simulink model "rate_change_filters_txrx_2ch"  (Simulink 8.0)
settings: Solver=VariableStepDiscrete  SolverMode=SingleTasking  StartTime=0.0  StopTime=1e3  RelTol=1e-3
InitFcn:
  | rate_change_filters_init
StartFcn:
  | rate_change_filters_init
values from neighbouring files (symbols this model uses):
  h32_rs = h32    [rate_change_filters_init.m]
  h64_rs = permute(reshape(h64(1:64),4,4,4),[2 1 3])    [rate_change_filters_init.m]
undefined symbols (not defined in the file or in its folder): gcbh, xlBlockLoadCallback, xlGetNormalizedPeriod
libraries: xbsIndex_r4 x519, simulink x4, xbsEDKLib_r4 x1
(part 3 of 4)

== system rate_change_filters_txrx_2ch/Tx Path ==
  2-Ch Interp A : Subsystem
  2-Ch Interp B : Subsystem
  Add : Sum  Inputs=+-
  Add1 : Sum  Inputs=+-
  Chirp : Subsystem
  Chirp1 : Subsystem
  Down Sample{1..4} (4 alike) : xbsIndex_r4/Down Sample  sample_ratio=8  sample_phase="Last Value of Frame  (most efficient)"  en=off  latency=1  dbl_ovrd=off  block_type=dsamp
      settings: xl_area=[8 16 0 0 0 0 0]  block_version=9.1.01
  Integer Delay : Delay  DelayLength=13*2  InputProcessing=Inherited
  Integer Delay1 : Delay  DelayLength=13*2  InputProcessing=Inherited
  Terminator1 : Terminator
  Terminator3 : Terminator
  Tx Scope : Scope  NumInputPorts=8
      settings: TickLabels=on  TimeRange=1000  YMin=-1~-1~-1~-1~-1~-1~-1~-1  YMax=1~1~1~1~1~1~1~1
  TxA_I_10M : xbsIndex_r4/Gateway In  gui_display_data_type=Fixed-point  arith_type="Signed  (2's comp)"  n_bits=16  bin_pt=15  preci_type=Single  exp_width=8  frac_width=24  quantization="Round  (unbiased: +/- Inf)"  overflow=Flag as error  period=1/2  dbl_ovrd=off  timing_constraint=None  locs_specified=off  LOCs={}  UseAsADC=off  ADCChannel='1'  inherit_from_input=off  hdl_port=on  block_type=gatewayin
      settings: infoedit="Gateway in block.  Converts inputs of type Simulink integer, double and fixed point to  Xilinx fixed point type.<P><P>Hardware notes:  In hardware these blocks become top level input ports."  xl_area=[0 0 0 0 16 0 0]  block_version=8.2.01
  TxA_I_40M : xbsIndex_r4/Gateway Out  inherit_from_input=off  hdl_port=on  timing_constraint=None  locs_specified=off  LOCs={}  UseAsDAC=off  DACChannel='1'  block_type=gatewayout
      settings: infoedit="Gateway out block.  Converts Xilinx fixed point inputs into ouputs of type Simulink integer, double, or fixed point.<P><P>Hardware notes:  In hardware these blocks become top level output ports or are discarded, depending on how they are configured."  xl_area=[0 0 0 0 16 0 0]  block_version=8.2.01
  TxA_Q_10M : xbsIndex_r4/Gateway In  gui_display_data_type=Fixed-point  arith_type="Signed  (2's comp)"  n_bits=16  bin_pt=15  preci_type=Single  exp_width=8  frac_width=24  quantization="Round  (unbiased: +/- Inf)"  overflow=Flag as error  period=1/2  dbl_ovrd=off  timing_constraint=None  locs_specified=off  LOCs={}  UseAsADC=off  ADCChannel='1'  inherit_from_input=off  hdl_port=on  block_type=gatewayin
      settings: infoedit="Gateway in block.  Converts inputs of type Simulink integer, double and fixed point to  Xilinx fixed point type.<P><P>Hardware notes:  In hardware these blocks become top level input ports."  xl_area=[0 0 0 0 16 0 0]  block_version=8.2.01
  TxA_Q_40M : xbsIndex_r4/Gateway Out  inherit_from_input=off  hdl_port=on  timing_constraint=None  locs_specified=off  LOCs={}  UseAsDAC=off  DACChannel='1'  block_type=gatewayout
      settings: infoedit="Gateway out block.  Converts Xilinx fixed point inputs into ouputs of type Simulink integer, double, or fixed point.<P><P>Hardware notes:  In hardware these blocks become top level output ports or are discarded, depending on how they are configured."  xl_area=[0 0 0 0 16 0 0]  block_version=8.2.01
  TxB_I_10M : xbsIndex_r4/Gateway In  gui_display_data_type=Fixed-point  arith_type="Signed  (2's comp)"  n_bits=16  bin_pt=15  preci_type=Single  exp_width=8  frac_width=24  quantization="Round  (unbiased: +/- Inf)"  overflow=Flag as error  period=1/2  dbl_ovrd=off  timing_constraint=None  locs_specified=off  LOCs={}  UseAsADC=off  ADCChannel='1'  inherit_from_input=off  hdl_port=on  block_type=gatewayin
      settings: infoedit="Gateway in block.  Converts inputs of type Simulink integer, double and fixed point to  Xilinx fixed point type.<P><P>Hardware notes:  In hardware these blocks become top level input ports."  xl_area=[0 0 0 0 16 0 0]  block_version=8.2.01
  TxB_I_40M : xbsIndex_r4/Gateway Out  inherit_from_input=off  hdl_port=on  timing_constraint=None  locs_specified=off  LOCs={}  UseAsDAC=off  DACChannel='1'  block_type=gatewayout
      settings: infoedit="Gateway out block.  Converts Xilinx fixed point inputs into ouputs of type Simulink integer, double, or fixed point.<P><P>Hardware notes:  In hardware these blocks become top level output ports or are discarded, depending on how they are configured."  xl_area=[0 0 0 0 16 0 0]  block_version=8.2.01
  TxB_Q_10M : xbsIndex_r4/Gateway In  gui_display_data_type=Fixed-point  arith_type="Signed  (2's comp)"  n_bits=16  bin_pt=15  preci_type=Single  exp_width=8  frac_width=24  quantization="Round  (unbiased: +/- Inf)"  overflow=Flag as error  period=1/2  dbl_ovrd=off  timing_constraint=None  locs_specified=off  LOCs={}  UseAsADC=off  ADCChannel='1'  inherit_from_input=off  hdl_port=on  block_type=gatewayin
      settings: infoedit="Gateway in block.  Converts inputs of type Simulink integer, double and fixed point to  Xilinx fixed point type.<P><P>Hardware notes:  In hardware these blocks become top level input ports."  xl_area=[0 0 0 0 16 0 0]  block_version=8.2.01
  TxB_Q_40M : xbsIndex_r4/Gateway Out  inherit_from_input=off  hdl_port=on  timing_constraint=None  locs_specified=off  LOCs={}  UseAsDAC=off  DACChannel='1'  block_type=gatewayout
      settings: infoedit="Gateway out block.  Converts Xilinx fixed point inputs into ouputs of type Simulink integer, double, or fixed point.<P><P>Hardware notes:  In hardware these blocks become top level output ports or are discarded, depending on how they are configured."  xl_area=[0 0 0 0 16 0 0]  block_version=8.2.01
  Up Sample{,1..3} (4 alike) : xbsIndex_r4/Up Sample  sample_ratio=2  copy_samples=on  en=off  latency=0  dbl_ovrd=off  block_type=usamp
      settings: infoedit="Up samples input data.  Inserted values  can be zeros or copies of the most recent input sample.<P><P>Hardware notes: No hardware is needed if inserted values are copies of the input sample; otherwise, a mux and single bit flip-flop are used."  xl_area=[0 0 0 0 0 0 0]  block_version=10.1.3
  wires:
  TxA_I_10M/1 -> Down Sample2/1
  TxA_Q_10M/1 -> Down Sample1/1
  TxB_I_10M/1 -> Down Sample3/1
  TxB_Q_10M/1 -> Down Sample4/1
  Down Sample2/1 -> 2-Ch Interp A/1(XA)
  Chirp/1(Out1) -> TxA_I_10M/1, TxB_I_10M/1, Tx Scope/1
  Integer Delay/1 -> Tx Scope/2, Add/1
  Add/1 -> Tx Scope/4
  Down Sample1/1 -> 2-Ch Interp A/2(XB)
  Chirp1/1(Out1) -> TxA_Q_10M/1, TxB_Q_10M/1, Tx Scope/5
  Add1/1 -> Tx Scope/8
  Down Sample3/1 -> 2-Ch Interp B/1(XA)
  Down Sample4/1 -> 2-Ch Interp B/2(XB)
  2-Ch Interp A/1(YA) -> Up Sample/1
  2-Ch Interp A/2(YB) -> Up Sample1/1
  2-Ch Interp B/1(YA) -> Up Sample2/1
  2-Ch Interp B/2(YB) -> Up Sample3/1
  TxA_I_40M/1 -> Integer Delay/1
  ? -> Tx Scope/3, Add/2
  TxA_Q_40M/1 -> Integer Delay1/1
  Integer Delay1/1 -> Tx Scope/6, Add1/1
  ? -> Tx Scope/7, Add1/2
  TxB_I_40M/1 -> Terminator3/1
  TxB_Q_40M/1 -> Terminator1/1
  Up Sample/1 -> TxA_I_40M/1
  Up Sample1/1 -> TxA_Q_40M/1
  Up Sample2/1 -> TxB_I_40M/1
  Up Sample3/1 -> TxB_Q_40M/1

== system rate_change_filters_txrx_2ch/Control & Coefficients/Rx Coefficients ==
  Addr : Inport
  ROM 0 : xbsIndex_r4/ROM  depth=4  initVector=h64_rs([1:4]+0)  distributed_mem=Distributed memory  rst=off  init_reg=0  en=off  latency=1  gui_display_data_type=Fixed-point  arith_type="Signed  (2's comp)"  n_bits=18  bin_pt=17  preci_type=Single  exp_width=8  frac_width=24  dbl_ovrd=off  optimize=Area  use_rpm=off  block_type=sprom
      settings: xl_area=[9 18 0 18 0 0 0]
  ROM 1 : xbsIndex_r4/ROM  depth=4  initVector=h64_rs([1:4]+4)  distributed_mem=Distributed memory  rst=off  init_reg=0  en=off  latency=1  gui_display_data_type=Fixed-point  arith_type="Signed  (2's comp)"  n_bits=18  bin_pt=17  preci_type=Single  exp_width=8  frac_width=24  dbl_ovrd=off  optimize=Area  use_rpm=off  block_type=sprom
      settings: xl_area=[9 18 0 18 0 0 0]
  ROM 10 : xbsIndex_r4/ROM  depth=4  initVector=h64_rs([1:4]+40)  distributed_mem=Distributed memory  rst=off  init_reg=0  en=off  latency=1  gui_display_data_type=Fixed-point  arith_type="Signed  (2's comp)"  n_bits=18  bin_pt=17  preci_type=Single  exp_width=8  frac_width=24  dbl_ovrd=off  optimize=Area  use_rpm=off  block_type=sprom
      settings: xl_area=[9 18 0 17 0 0 0]
  ROM 11 : xbsIndex_r4/ROM  depth=4  initVector=h64_rs([1:4]+44)  distributed_mem=Distributed memory  rst=off  init_reg=0  en=off  latency=1  gui_display_data_type=Fixed-point  arith_type="Signed  (2's comp)"  n_bits=18  bin_pt=17  preci_type=Single  exp_width=8  frac_width=24  dbl_ovrd=off  optimize=Area  use_rpm=off  block_type=sprom
      settings: xl_area=[9 18 0 17 0 0 0]
  ROM 12 : xbsIndex_r4/ROM  depth=4  initVector=h64_rs([1:4]+48)  distributed_mem=Distributed memory  rst=off  init_reg=0  en=off  latency=1  gui_display_data_type=Fixed-point  arith_type="Signed  (2's comp)"  n_bits=18  bin_pt=17  preci_type=Single  exp_width=8  frac_width=24  dbl_ovrd=off  optimize=Area  use_rpm=off  block_type=sprom
      settings: xl_area=[9 18 0 17 0 0 0]
  ROM 13 : xbsIndex_r4/ROM  depth=4  initVector=h64_rs([1:4]+52)  distributed_mem=Distributed memory  rst=off  init_reg=0  en=off  latency=1  gui_display_data_type=Fixed-point  arith_type="Signed  (2's comp)"  n_bits=18  bin_pt=17  preci_type=Single  exp_width=8  frac_width=24  dbl_ovrd=off  optimize=Area  use_rpm=off  block_type=sprom
      settings: xl_area=[9 18 0 18 0 0 0]
  ROM 14 : xbsIndex_r4/ROM  depth=4  initVector=h64_rs([1:4]+56)  distributed_mem=Distributed memory  rst=off  init_reg=0  en=off  latency=1  gui_display_data_type=Fixed-point  arith_type="Signed  (2's comp)"  n_bits=18  bin_pt=17  preci_type=Single  exp_width=8  frac_width=24  dbl_ovrd=off  optimize=Area  use_rpm=off  block_type=sprom
      settings: xl_area=[9 18 0 18 0 0 0]
  ROM 15 : xbsIndex_r4/ROM  depth=4  initVector=h64_rs([1:4]+60)  distributed_mem=Distributed memory  rst=off  init_reg=0  en=off  latency=1  gui_display_data_type=Fixed-point  arith_type="Signed  (2's comp)"  n_bits=18  bin_pt=17  preci_type=Single  exp_width=8  frac_width=24  dbl_ovrd=off  optimize=Area  use_rpm=off  block_type=sprom
      settings: xl_area=[9 18 0 18 0 0 0]
  ROM 2 : xbsIndex_r4/ROM  depth=4  initVector=h64_rs([1:4]+8)  distributed_mem=Distributed memory  rst=off  init_reg=0  en=off  latency=1  gui_display_data_type=Fixed-point  arith_type="Signed  (2's comp)"  n_bits=18  bin_pt=17  preci_type=Single  exp_width=8  frac_width=24  dbl_ovrd=off  optimize=Area  use_rpm=off  block_type=sprom
      settings: xl_area=[9 18 0 18 0 0 0]
  ROM 3 : xbsIndex_r4/ROM  depth=4  initVector=h64_rs([1:4]+12)  distributed_mem=Distributed memory  rst=off  init_reg=0  en=off  latency=1  gui_display_data_type=Fixed-point  arith_type="Signed  (2's comp)"  n_bits=18  bin_pt=17  preci_type=Single  exp_width=8  frac_width=24  dbl_ovrd=off  optimize=Area  use_rpm=off  block_type=sprom
      settings: xl_area=[9 18 0 17 0 0 0]
  ROM 4 : xbsIndex_r4/ROM  depth=4  initVector=h64_rs([1:4]+16)  distributed_mem=Distributed memory  rst=off  init_reg=0  en=off  latency=1  gui_display_data_type=Fixed-point  arith_type="Signed  (2's comp)"  n_bits=18  bin_pt=17  preci_type=Single  exp_width=8  frac_width=24  dbl_ovrd=off  optimize=Area  use_rpm=off  block_type=sprom
      settings: xl_area=[9 18 0 17 0 0 0]
  ROM 5 : xbsIndex_r4/ROM  depth=4  initVector=h64_rs([1:4]+20)  distributed_mem=Distributed memory  rst=off  init_reg=0  en=off  latency=1  gui_display_data_type=Fixed-point  arith_type="Signed  (2's comp)"  n_bits=18  bin_pt=17  preci_type=Single  exp_width=8  frac_width=24  dbl_ovrd=off  optimize=Area  use_rpm=off  block_type=sprom
      settings: xl_area=[9 18 0 17 0 0 0]
  ROM 6 : xbsIndex_r4/ROM  depth=4  initVector=h64_rs([1:4]+24)  distributed_mem=Distributed memory  rst=off  init_reg=0  en=off  latency=1  gui_display_data_type=Fixed-point  arith_type="Signed  (2's comp)"  n_bits=18  bin_pt=17  preci_type=Single  exp_width=8  frac_width=24  dbl_ovrd=off  optimize=Area  use_rpm=off  block_type=sprom
      settings: xl_area=[9 18 0 18 0 0 0]
  ROM 7 : xbsIndex_r4/ROM  depth=4  initVector=h64_rs([1:4]+28)  distributed_mem=Distributed memory  rst=off  init_reg=0  en=off  latency=1  gui_display_data_type=Fixed-point  arith_type="Signed  (2's comp)"  n_bits=18  bin_pt=17  preci_type=Single  exp_width=8  frac_width=24  dbl_ovrd=off  optimize=Area  use_rpm=off  block_type=sprom
      settings: xl_area=[9 18 0 16 0 0 0]
  ROM 8 : xbsIndex_r4/ROM  depth=4  initVector=h64_rs([1:4]+32)  distributed_mem=Distributed memory  rst=off  init_reg=0  en=off  latency=1  gui_display_data_type=Fixed-point  arith_type="Signed  (2's comp)"  n_bits=18  bin_pt=17  preci_type=Single  exp_width=8  frac_width=24  dbl_ovrd=off  optimize=Area  use_rpm=off  block_type=sprom
      settings: xl_area=[9 18 0 16 0 0 0]
  ROM 9 : xbsIndex_r4/ROM  depth=4  initVector=h64_rs([1:4]+36)  distributed_mem=Distributed memory  rst=off  init_reg=0  en=off  latency=1  gui_display_data_type=Fixed-point  arith_type="Signed  (2's comp)"  n_bits=18  bin_pt=17  preci_type=Single  exp_width=8  frac_width=24  dbl_ovrd=off  optimize=Area  use_rpm=off  block_type=sprom
      settings: xl_area=[9 18 0 18 0 0 0]
  tag scope: ROM_0=global, ROM_10=global, ROM_11=global, ROM_12=global, ROM_13=global, ROM_14=global, ROM_15=global, ROM_1=global, ROM_2=global, ROM_3=global, ROM_4=global, ROM_5=global, ROM_6=global, ROM_7=global, ROM_8=global, ROM_9=global
  wires:
  Addr/1 -> ROM 0/1, ROM 14/1, ROM 15/1, ROM 13/1, ROM 12/1, ROM 11/1, ROM 10/1, ROM 9/1, ROM 8/1, ROM 7/1, ROM 6/1, ROM 5/1, ROM 4/1, ROM 3/1, ROM 2/1, ROM 1/1
  ROM 15/1 -> [ROM_15]
  ROM 14/1 -> [ROM_14]
  ROM 13/1 -> [ROM_13]
  ROM 12/1 -> [ROM_12]
  ROM 11/1 -> [ROM_11]
  ROM 10/1 -> [ROM_10]
  ROM 9/1 -> [ROM_9]
  ROM 8/1 -> [ROM_8]
  ROM 7/1 -> [ROM_7]
  ROM 6/1 -> [ROM_6]
  ROM 5/1 -> [ROM_5]
  ROM 4/1 -> [ROM_4]
  ROM 3/1 -> [ROM_3]
  ROM 2/1 -> [ROM_2]
  ROM 1/1 -> [ROM_1]
  ROM 0/1 -> [ROM_0]

== system rate_change_filters_txrx_2ch/Control & Coefficients/Tx Coefficients ==
  Addr : Inport
  ROM 0 : xbsIndex_r4/ROM  depth=4  initVector=h32_rs([1:4]+0)  distributed_mem=Distributed memory  rst=off  init_reg=0  en=off  latency=1  gui_display_data_type=Fixed-point  arith_type="Signed  (2's comp)"  n_bits=18  bin_pt=17  preci_type=Single  exp_width=8  frac_width=24  dbl_ovrd=off  optimize=Area  use_rpm=off  block_type=sprom
      settings: xl_area=[9 18 0 18 0 0 0]
  ROM 1 : xbsIndex_r4/ROM  depth=4  initVector=h32_rs([1:4]+4)  distributed_mem=Distributed memory  rst=off  init_reg=0  en=off  latency=1  gui_display_data_type=Fixed-point  arith_type="Signed  (2's comp)"  n_bits=18  bin_pt=17  preci_type=Single  exp_width=8  frac_width=24  dbl_ovrd=off  optimize=Area  use_rpm=off  block_type=sprom
      settings: xl_area=[9 18 0 14 0 0 0]
  ROM 2 : xbsIndex_r4/ROM  depth=4  initVector=h32_rs([1:4]+8)  distributed_mem=Distributed memory  rst=off  init_reg=0  en=off  latency=1  gui_display_data_type=Fixed-point  arith_type="Signed  (2's comp)"  n_bits=18  bin_pt=17  preci_type=Single  exp_width=8  frac_width=24  dbl_ovrd=off  optimize=Area  use_rpm=off  block_type=sprom
      settings: xl_area=[9 18 0 17 0 0 0]
  ROM 3 : xbsIndex_r4/ROM  depth=4  initVector=h32_rs([1:4]+12)  distributed_mem=Distributed memory  rst=off  init_reg=0  en=off  latency=1  gui_display_data_type=Fixed-point  arith_type="Signed  (2's comp)"  n_bits=18  bin_pt=17  preci_type=Single  exp_width=8  frac_width=24  dbl_ovrd=off  optimize=Area  use_rpm=off  block_type=sprom
      settings: xl_area=[9 18 0 16 0 0 0]
  ROM 4 : xbsIndex_r4/ROM  depth=4  initVector=h32_rs([1:4]+16)  distributed_mem=Distributed memory  rst=off  init_reg=0  en=off  latency=1  gui_display_data_type=Fixed-point  arith_type="Signed  (2's comp)"  n_bits=18  bin_pt=17  preci_type=Single  exp_width=8  frac_width=24  dbl_ovrd=off  optimize=Area  use_rpm=off  block_type=sprom
      settings: xl_area=[9 18 0 16 0 0 0]
  ROM 5 : xbsIndex_r4/ROM  depth=4  initVector=h32_rs([1:4]+20)  distributed_mem=Distributed memory  rst=off  init_reg=0  en=off  latency=1  gui_display_data_type=Fixed-point  arith_type="Signed  (2's comp)"  n_bits=18  bin_pt=17  preci_type=Single  exp_width=8  frac_width=24  dbl_ovrd=off  optimize=Area  use_rpm=off  block_type=sprom
      settings: xl_area=[9 18 0 17 0 0 0]
  ROM 6 : xbsIndex_r4/ROM  depth=4  initVector=h32_rs([1:4]+24)  distributed_mem=Distributed memory  rst=off  init_reg=0  en=off  latency=1  gui_display_data_type=Fixed-point  arith_type="Signed  (2's comp)"  n_bits=18  bin_pt=17  preci_type=Single  exp_width=8  frac_width=24  dbl_ovrd=off  optimize=Area  use_rpm=off  block_type=sprom
      settings: xl_area=[9 18 0 14 0 0 0]
  ROM 7 : xbsIndex_r4/ROM  depth=4  initVector=h32_rs([1:4]+28)  distributed_mem=Distributed memory  rst=off  init_reg=0  en=off  latency=1  gui_display_data_type=Fixed-point  arith_type="Signed  (2's comp)"  n_bits=18  bin_pt=17  preci_type=Single  exp_width=8  frac_width=24  dbl_ovrd=off  optimize=Area  use_rpm=off  block_type=sprom
      settings: xl_area=[9 18 0 18 0 0 0]
  tag scope: TX_ROM_0=global, TX_ROM_1=global, TX_ROM_2=global, TX_ROM_3=global, TX_ROM_4=global, TX_ROM_5=global, TX_ROM_6=global, TX_ROM_7=global
  wires:
  ROM 0/1 -> [TX_ROM_0]
  ROM 1/1 -> [TX_ROM_1]
  ROM 2/1 -> [TX_ROM_2]
  ROM 3/1 -> [TX_ROM_3]
  ROM 4/1 -> [TX_ROM_4]
  ROM 5/1 -> [TX_ROM_5]
  ROM 6/1 -> [TX_ROM_6]
  ROM 7/1 -> [TX_ROM_7]
  Addr/1 -> ROM 1/1, ROM 2/1, ROM 3/1, ROM 4/1, ROM 5/1, ROM 6/1, ROM 7/1, ROM 0/1

== system rate_change_filters_txrx_2ch/Rx Path/2-Ch Decimation A ==
  note: This convert will overflow, but never for
      | the output samples that are actually
      | captured by the next register.
  note: Need a pipeline stage here to meet 80MHz timing when using non-DSP48 mults in V4.
      | Need double-delays to keep everything lined up
      | when processing two interleaved sample streams.
  XA : Inport
  XB : Inport  Port=2
  Accumulator : xbsIndex_r4/Accumulator  operation=Add  n_bits=32  overflow=Flag as error  scale=1  rst=on  infoeditControl=reset for floating point data type must be asserted for a minimum of 2 cycles  hasbypass=on  en=off  latency=0  dbl_ovrd=off  msb_inp=100  msb=100  lsb=-100  use_behavioral_HDL=on  implementation=Fabric  block_type=accum
      settings: infoedit="Adder or subtractor-based accumulator.   Output type and binary point position match the input.<P><P>Hardware notes: When \"Reinitialize with input 'b' on reset\" is selected, the accumulator is forced to run at the system rate even if the input 'b' is running at a slower rate."  xl_area=[17 33 0 32 0 0 0]  block_version=9.1.01
  Accumulator1 : xbsIndex_r4/Accumulator  operation=Add  n_bits=32  overflow=Flag as error  scale=1  rst=on  infoeditControl=reset for floating point data type must be asserted for a minimum of 2 cycles  hasbypass=on  en=off  latency=0  dbl_ovrd=off  msb_inp=100  msb=100  lsb=-100  use_behavioral_HDL=on  implementation=Fabric  block_type=accum
      settings: infoedit="Adder or subtractor-based accumulator.   Output type and binary point position match the input.<P><P>Hardware notes: When \"Reinitialize with input 'b' on reset\" is selected, the accumulator is forced to run at the system rate even if the input 'b' is running at a slower rate."  xl_area=[17 33 0 32 0 0 0]  block_version=9.1.01
  Adders : Subsystem
  Constant : xbsIndex_r4/Constant  const=3  gui_display_data_type=Fixed-point  arith_type=Unsigned  n_bits=3  bin_pt=0  preci_type=Single  exp_width=8  frac_width=24  explicit_period=off  period=1  equ=P=C  opselect=C  inp2=PCIN>>17  opr=+  inp1=P  carry=CIN  dbl_ovrd=off  block_type=constant
      settings: block_version=9.1.01
  Convert : xbsIndex_r4/Convert  gui_display_data_type=Fixed-point  arith_type="Signed  (2's comp)"  n_bits=14  bin_pt=13  float_type=Single  exp_bits=8  fraction_bits=24  quantization="Round  (unbiased: +/- Inf)"  overflow=Wrap  en=off  latency=0  dbl_ovrd=off  pipeline=off  block_type=convert
      settings: xl_area=[11 0 0 18 0 0 0]  block_version=10.1.3
  Convert1 : xbsIndex_r4/Convert  gui_display_data_type=Fixed-point  arith_type="Signed  (2's comp)"  n_bits=14  bin_pt=13  float_type=Single  exp_bits=8  fraction_bits=24  quantization="Round  (unbiased: +/- Inf)"  overflow=Wrap  en=off  latency=0  dbl_ovrd=off  pipeline=off  block_type=convert
      settings: xl_area=[11 0 0 18 0 0 0]  block_version=10.1.3
  Delay1 : xbsIndex_r4/Delay  rst=off  infoeditControl=Selection of Reset will increase slice count due to use of real FFs and instead of SRLs  en=off  latency=0  dbl_ovrd=off  reg_retiming=off  block_type=delay
      settings: xl_area=[0 0 0 0 0 0 0]  block_version=9.1.01
  Delay16 : xbsIndex_r4/Delay  rst=off  infoeditControl=Selection of Reset will increase slice count due to use of real FFs and instead of SRLs  en=off  latency=0  dbl_ovrd=off  reg_retiming=off  block_type=delay
      settings: xl_area=[0 0 0 0 0 0 0]  block_version=9.1.01
  Delays : Subsystem
  Down Sample : xbsIndex_r4/Down Sample  sample_ratio=4  sample_phase=First Value of Frame  en=off  latency=0  dbl_ovrd=off  block_type=dsamp
      settings: xl_area=[15 15 0 14 0 0 0]  block_version=9.1.01
  Down Sample1 : xbsIndex_r4/Down Sample  sample_ratio=4  sample_phase=First Value of Frame  en=off  latency=0  dbl_ovrd=off  block_type=dsamp
      settings: xl_area=[15 15 0 14 0 0 0]  block_version=9.1.01
  ROMS & Mults : Subsystem
  Register : xbsIndex_r4/Register  init=0  rst=off  en=on  dbl_ovrd=off  block_type=register
      settings: xl_area=[7 14 0 0 0 0 0]  block_version=9.1.01
  Register1 : xbsIndex_r4/Register  init=0  rst=off  en=on  dbl_ovrd=off  block_type=register
      settings: xl_area=[7 14 0 0 0 0 0]  block_version=9.1.01
  Relational : xbsIndex_r4/Relational  mode=a=b  en=off  latency=0  dbl_ovrd=off  block_type=relational
      settings: xl_area=[1 0 0 2 0 0 0]  block_version=9.1.01
  Sample RAMs : Subsystem
  Scale : xbsIndex_r4/Scale  scale_factor=-2  dbl_ovrd=off  block_type=scale
      settings: infoedit=Scales input by a power of two by adjusting the binary point position.<P><P>Hardware notes: In hardware this block costs nothing.  block_version=10.1.3
  Scale1 : xbsIndex_r4/Scale  scale_factor=-2  dbl_ovrd=off  block_type=scale
      settings: infoedit=Scales input by a power of two by adjusting the binary point position.<P><P>Hardware notes: In hardware this block costs nothing.  block_version=10.1.3
  TDD : xbsIndex_r4/Time Division Demultiplexer  frame_pattern=ones(1,2)  impl_style=Multiple Channel  vin=off  dbl_ovrd=off  explicit_period=off  period=1  block_type=tdd
      settings: infoedit=Samples presented at the input are selected and down-sampled according to the frame sampling pattern specified. The sampled input is presented either as a single or multiple channel at the output.  xl_area=[42 84 0 0 0 0 0]  block_version=9.1.01
  YA : Outport
  YB : Outport  Port=2
  wires:
  ROMS & Mults/8(Out8) -> Adders/8(In8)
  ROMS & Mults/7(Out7) -> Adders/7(In7)
  ROMS & Mults/6(Out6) -> Adders/6(In6)
  ROMS & Mults/5(Out5) -> Adders/5(In5)
  ROMS & Mults/4(Out4) -> Adders/4(In4)
  ROMS & Mults/3(Out3) -> Adders/3(In3)
  ROMS & Mults/2(Out2) -> Adders/2(In2)
  ROMS & Mults/1(Out1) -> Adders/1(In1)
  ROMS & Mults/16(Out16) -> Adders/16(In16)
  ROMS & Mults/15(Out15) -> Adders/15(In15)
  ROMS & Mults/14(Out14) -> Adders/14(In14)
  ROMS & Mults/13(Out13) -> Adders/13(In13)
  ROMS & Mults/12(Out12) -> Adders/12(In12)
  ROMS & Mults/11(Out11) -> Adders/11(In11)
  ROMS & Mults/10(Out10) -> Adders/10(In10)
  ROMS & Mults/9(Out9) -> Adders/9(In9)
  Register/1 -> Down Sample/1
  Down Sample/1 -> YB/1
  Constant/1 -> Relational/1
  Accumulator/1 -> Scale/1
  [CoefAddr] -> Delay16/1, Delay1/1
  Scale/1 -> Convert/1
  Convert/1 -> Register/1
  XA/1 -> Sample RAMs/1(XA)
  XB/1 -> Sample RAMs/2(XB)
  Accumulator1/1 -> Scale1/1
  Scale1/1 -> Convert1/1
  Convert1/1 -> Register1/1
  Register1/1 -> Down Sample1/1
  Down Sample1/1 -> YA/1
  Adders/1(Out1) -> TDD/1
  TDD/1 -> Accumulator1/1
  TDD/2 -> Accumulator/1
  Relational/1 -> Accumulator1/2, Accumulator/2, Register1/2, Register/2
  Sample RAMs/1(Out1) -> Delays/1(In1)
  Sample RAMs/2(Out2) -> Delays/2(In2)
  Sample RAMs/3(Out3) -> Delays/3(In3)
  Sample RAMs/4(Out4) -> Delays/4(In4)
  Sample RAMs/5(Out5) -> Delays/5(In5)
  Sample RAMs/6(Out6) -> Delays/6(In6)
  Sample RAMs/7(Out7) -> Delays/7(In7)
  Sample RAMs/8(Out8) -> Delays/8(In8)
  Sample RAMs/9(Out9) -> Delays/9(In9)
  Sample RAMs/10(Out10) -> Delays/10(In10)
  Sample RAMs/11(Out11) -> Delays/11(In11)
  Sample RAMs/12(Out12) -> Delays/12(In12)
  Sample RAMs/13(Out13) -> Delays/13(In13)
  Sample RAMs/14(Out14) -> Delays/14(In14)
  Sample RAMs/15(Out15) -> Delays/15(In15)
  Sample RAMs/16(Out16) -> Delays/16(In16)
  Delay16/1 -> Sample RAMs/3(Addr)
  Delay1/1 -> Relational/2
  Delays/1(Out1) -> ROMS & Mults/1(In1)
  Delays/2(Out2) -> ROMS & Mults/2(In2)
  Delays/3(Out3) -> ROMS & Mults/3(In3)
  Delays/4(Out4) -> ROMS & Mults/4(In4)
  Delays/5(Out5) -> ROMS & Mults/5(In5)
  Delays/6(Out6) -> ROMS & Mults/6(In6)
  Delays/7(Out7) -> ROMS & Mults/7(In7)
  Delays/8(Out8) -> ROMS & Mults/8(In8)
  Delays/9(Out9) -> ROMS & Mults/9(In9)
  Delays/10(Out10) -> ROMS & Mults/10(In10)
  Delays/11(Out11) -> ROMS & Mults/11(In11)
  Delays/12(Out12) -> ROMS & Mults/12(In12)
  Delays/13(Out13) -> ROMS & Mults/13(In13)
  Delays/14(Out14) -> ROMS & Mults/14(In14)
  Delays/15(Out15) -> ROMS & Mults/15(In15)
  Delays/16(Out16) -> ROMS & Mults/16(In16)

== system rate_change_filters_txrx_2ch/Rx Path/2-Ch Decimation B ==
  note: Need a pipeline stage here to meet 80MHz timing when using non-DSP48 mults in V4.
      | Need double-delays to keep everything lined up
      | when processing two interleaved sample streams.
  note: This convert will overflow, but never for
      | the output samples that are actually
      | captured by the next register.
  XA : Inport
  XB : Inport  Port=2
  Accumulator : xbsIndex_r4/Accumulator  operation=Add  n_bits=32  overflow=Flag as error  scale=1  rst=on  infoeditControl=reset for floating point data type must be asserted for a minimum of 2 cycles  hasbypass=on  en=off  latency=0  dbl_ovrd=off  msb_inp=100  msb=100  lsb=-100  use_behavioral_HDL=on  implementation=Fabric  block_type=accum
      settings: infoedit="Adder or subtractor-based accumulator.   Output type and binary point position match the input.<P><P>Hardware notes: When \"Reinitialize with input 'b' on reset\" is selected, the accumulator is forced to run at the system rate even if the input 'b' is running at a slower rate."  xl_area=[17 33 0 32 0 0 0]  block_version=9.1.01
  Accumulator1 : xbsIndex_r4/Accumulator  operation=Add  n_bits=32  overflow=Flag as error  scale=1  rst=on  infoeditControl=reset for floating point data type must be asserted for a minimum of 2 cycles  hasbypass=on  en=off  latency=0  dbl_ovrd=off  msb_inp=100  msb=100  lsb=-100  use_behavioral_HDL=on  implementation=Fabric  block_type=accum
      settings: infoedit="Adder or subtractor-based accumulator.   Output type and binary point position match the input.<P><P>Hardware notes: When \"Reinitialize with input 'b' on reset\" is selected, the accumulator is forced to run at the system rate even if the input 'b' is running at a slower rate."  xl_area=[17 33 0 32 0 0 0]  block_version=9.1.01
  Adders : Subsystem
  Constant : xbsIndex_r4/Constant  const=3  gui_display_data_type=Fixed-point  arith_type=Unsigned  n_bits=3  bin_pt=0  preci_type=Single  exp_width=8  frac_width=24  explicit_period=off  period=1  equ=P=C  opselect=C  inp2=PCIN>>17  opr=+  inp1=P  carry=CIN  dbl_ovrd=off  block_type=constant
      settings: block_version=9.1.01
  Convert : xbsIndex_r4/Convert  gui_display_data_type=Fixed-point  arith_type="Signed  (2's comp)"  n_bits=14  bin_pt=13  float_type=Single  exp_bits=8  fraction_bits=24  quantization="Round  (unbiased: +/- Inf)"  overflow=Wrap  en=off  latency=0  dbl_ovrd=off  pipeline=off  block_type=convert
      settings: xl_area=[11 0 0 18 0 0 0]  block_version=10.1.3
  Convert1 : xbsIndex_r4/Convert  gui_display_data_type=Fixed-point  arith_type="Signed  (2's comp)"  n_bits=14  bin_pt=13  float_type=Single  exp_bits=8  fraction_bits=24  quantization="Round  (unbiased: +/- Inf)"  overflow=Wrap  en=off  latency=0  dbl_ovrd=off  pipeline=off  block_type=convert
      settings: xl_area=[11 0 0 18 0 0 0]  block_version=10.1.3
  Delay1 : xbsIndex_r4/Delay  rst=off  infoeditControl=Selection of Reset will increase slice count due to use of real FFs and instead of SRLs  en=off  latency=0  dbl_ovrd=off  reg_retiming=off  block_type=delay
      settings: xl_area=[0 0 0 0 0 0 0]  block_version=9.1.01
  Delay16 : xbsIndex_r4/Delay  rst=off  infoeditControl=Selection of Reset will increase slice count due to use of real FFs and instead of SRLs  en=off  latency=0  dbl_ovrd=off  reg_retiming=off  block_type=delay
      settings: xl_area=[0 0 0 0 0 0 0]  block_version=9.1.01
  Delays : Subsystem
  Down Sample : xbsIndex_r4/Down Sample  sample_ratio=4  sample_phase=First Value of Frame  en=off  latency=0  dbl_ovrd=off  block_type=dsamp
      settings: xl_area=[15 15 0 14 0 0 0]  block_version=9.1.01
  Down Sample1 : xbsIndex_r4/Down Sample  sample_ratio=4  sample_phase=First Value of Frame  en=off  latency=0  dbl_ovrd=off  block_type=dsamp
      settings: xl_area=[15 15 0 14 0 0 0]  block_version=9.1.01
  ROMS & Mults : Subsystem
  Register : xbsIndex_r4/Register  init=0  rst=off  en=on  dbl_ovrd=off  block_type=register
      settings: xl_area=[7 14 0 0 0 0 0]  block_version=9.1.01
  Register1 : xbsIndex_r4/Register  init=0  rst=off  en=on  dbl_ovrd=off  block_type=register
      settings: xl_area=[7 14 0 0 0 0 0]  block_version=9.1.01
  Relational : xbsIndex_r4/Relational  mode=a=b  en=off  latency=0  dbl_ovrd=off  block_type=relational
      settings: xl_area=[1 0 0 2 0 0 0]  block_version=9.1.01
  Sample RAMs : Subsystem
  Scale : xbsIndex_r4/Scale  scale_factor=-2  dbl_ovrd=off  block_type=scale
      settings: infoedit=Scales input by a power of two by adjusting the binary point position.<P><P>Hardware notes: In hardware this block costs nothing.  block_version=10.1.3
  Scale1 : xbsIndex_r4/Scale  scale_factor=-2  dbl_ovrd=off  block_type=scale
      settings: infoedit=Scales input by a power of two by adjusting the binary point position.<P><P>Hardware notes: In hardware this block costs nothing.  block_version=10.1.3
  TDD : xbsIndex_r4/Time Division Demultiplexer  frame_pattern=ones(1,2)  impl_style=Multiple Channel  vin=off  dbl_ovrd=off  explicit_period=off  period=1  block_type=tdd
      settings: infoedit=Samples presented at the input are selected and down-sampled according to the frame sampling pattern specified. The sampled input is presented either as a single or multiple channel at the output.  xl_area=[42 84 0 0 0 0 0]  block_version=9.1.01
  YA : Outport
  YB : Outport  Port=2
  wires:
  Delays/16(Out16) -> ROMS & Mults/16(In16)
  Delays/15(Out15) -> ROMS & Mults/15(In15)
  Delays/14(Out14) -> ROMS & Mults/14(In14)
  Delays/13(Out13) -> ROMS & Mults/13(In13)
  Delays/12(Out12) -> ROMS & Mults/12(In12)
  Delays/11(Out11) -> ROMS & Mults/11(In11)
  Delays/10(Out10) -> ROMS & Mults/10(In10)
  Delays/9(Out9) -> ROMS & Mults/9(In9)
  Delays/8(Out8) -> ROMS & Mults/8(In8)
  Delays/7(Out7) -> ROMS & Mults/7(In7)
  Delays/6(Out6) -> ROMS & Mults/6(In6)
  Delays/5(Out5) -> ROMS & Mults/5(In5)
  Delays/4(Out4) -> ROMS & Mults/4(In4)
  Delays/3(Out3) -> ROMS & Mults/3(In3)
  Delays/2(Out2) -> ROMS & Mults/2(In2)
  Delays/1(Out1) -> ROMS & Mults/1(In1)
  Delay1/1 -> Relational/2
  Delay16/1 -> Sample RAMs/3(Addr)
  Sample RAMs/16(Out16) -> Delays/16(In16)
  Sample RAMs/15(Out15) -> Delays/15(In15)
  Sample RAMs/14(Out14) -> Delays/14(In14)
  Sample RAMs/13(Out13) -> Delays/13(In13)
  Sample RAMs/12(Out12) -> Delays/12(In12)
  Sample RAMs/11(Out11) -> Delays/11(In11)
  Sample RAMs/10(Out10) -> Delays/10(In10)
  Sample RAMs/9(Out9) -> Delays/9(In9)
  Sample RAMs/8(Out8) -> Delays/8(In8)
  Sample RAMs/7(Out7) -> Delays/7(In7)
  Sample RAMs/6(Out6) -> Delays/6(In6)
  Sample RAMs/5(Out5) -> Delays/5(In5)
  Sample RAMs/4(Out4) -> Delays/4(In4)
  Sample RAMs/3(Out3) -> Delays/3(In3)
  Sample RAMs/2(Out2) -> Delays/2(In2)
  Sample RAMs/1(Out1) -> Delays/1(In1)
  Relational/1 -> Register/2, Register1/2, Accumulator/2, Accumulator1/2
  TDD/2 -> Accumulator/1
  TDD/1 -> Accumulator1/1
  Adders/1(Out1) -> TDD/1
  Down Sample1/1 -> YA/1
  Register1/1 -> Down Sample1/1
  Convert1/1 -> Register1/1
  Scale1/1 -> Convert1/1
  Accumulator1/1 -> Scale1/1
  XB/1 -> Sample RAMs/2(XB)
  XA/1 -> Sample RAMs/1(XA)
  Convert/1 -> Register/1
  Scale/1 -> Convert/1
  [CoefAddr] -> Delay1/1, Delay16/1
  Accumulator/1 -> Scale/1
  Constant/1 -> Relational/1
  Down Sample/1 -> YB/1
  Register/1 -> Down Sample/1
  ROMS & Mults/9(Out9) -> Adders/9(In9)
  ROMS & Mults/10(Out10) -> Adders/10(In10)
  ROMS & Mults/11(Out11) -> Adders/11(In11)
  ROMS & Mults/12(Out12) -> Adders/12(In12)
  ROMS & Mults/13(Out13) -> Adders/13(In13)
  ROMS & Mults/14(Out14) -> Adders/14(In14)
  ROMS & Mults/15(Out15) -> Adders/15(In15)
  ROMS & Mults/16(Out16) -> Adders/16(In16)
  ROMS & Mults/1(Out1) -> Adders/1(In1)
  ROMS & Mults/2(Out2) -> Adders/2(In2)
  ROMS & Mults/3(Out3) -> Adders/3(In3)
  ROMS & Mults/4(Out4) -> Adders/4(In4)
  ROMS & Mults/5(Out5) -> Adders/5(In5)
  ROMS & Mults/6(Out6) -> Adders/6(In6)
  ROMS & Mults/7(Out7) -> Adders/7(In7)
  ROMS & Mults/8(Out8) -> Adders/8(In8)

== system rate_change_filters_txrx_2ch/Rx Path/Chirp ==
  Chirp Signal : simulink/Sources/Chirp Signal  f1=0  T=512  f2=0.5
  Gain : Gain  Gain=0.99
  Out1 : Outport
  wires:
  Chirp Signal/1 -> Gain/1
  Gain/1 -> Out1/1

== system rate_change_filters_txrx_2ch/Rx Path/Chirp1 ==
  Chirp Signal : simulink/Sources/Chirp Signal  f1=0  T=512  f2=0.5
  Gain : Gain  Gain=-0.99
  Out1 : Outport
  wires:
  Gain/1 -> Out1/1
  Chirp Signal/1 -> Gain/1

== system rate_change_filters_txrx_2ch/Tx Path/2-Ch Interp A ==
  XA : Inport
  XB : Inport  Port=2
  Adders : Subsystem
  Mults & ROMs : Subsystem
  Sample RAMs : Subsystem
  TDD : xbsIndex_r4/Time Division Demultiplexer  frame_pattern=ones(1,2)  impl_style=Multiple Channel  vin=off  dbl_ovrd=off  explicit_period=off  period=1  block_type=tdd
      settings: infoedit=Samples presented at the input are selected and down-sampled according to the frame sampling pattern specified. The sampled input is presented either as a single or multiple channel at the output.  xl_area=[24 48 0 0 0 0 0]  block_version=9.1.01
  YA : Outport
  YB : Outport  Port=2
  wires:
  Mults & ROMs/8(Out8) -> Adders/8(In8)
  Mults & ROMs/7(Out7) -> Adders/7(In7)
  Mults & ROMs/6(Out6) -> Adders/6(In6)
  Mults & ROMs/5(Out5) -> Adders/5(In5)
  Mults & ROMs/4(Out4) -> Adders/4(In4)
  Mults & ROMs/3(Out3) -> Adders/3(In3)
  Mults & ROMs/2(Out2) -> Adders/2(In2)
  Mults & ROMs/1(Out1) -> Adders/1(In1)
  XA/1 -> Sample RAMs/1(A)
  XB/1 -> Sample RAMs/2(B)
  Sample RAMs/1(Out1) -> Mults & ROMs/1(In1)
  Sample RAMs/2(Out2) -> Mults & ROMs/2(In2)
  Sample RAMs/3(Out3) -> Mults & ROMs/3(In3)
  Sample RAMs/4(Out4) -> Mults & ROMs/4(In4)
  Sample RAMs/5(Out5) -> Mults & ROMs/5(In5)
  Sample RAMs/6(Out6) -> Mults & ROMs/6(In6)
  Sample RAMs/7(Out7) -> Mults & ROMs/7(In7)
  Sample RAMs/8(Out8) -> Mults & ROMs/8(In8)
  Adders/1(Out1) -> TDD/1
  TDD/1 -> YA/1
  TDD/2 -> YB/1

== system rate_change_filters_txrx_2ch/Tx Path/2-Ch Interp B ==
  XA : Inport
  XB : Inport  Port=2
  Adders : Subsystem
  Mults & ROMs : Subsystem
  Sample RAMs : Subsystem
  TDD : xbsIndex_r4/Time Division Demultiplexer  frame_pattern=ones(1,2)  impl_style=Multiple Channel  vin=off  dbl_ovrd=off  explicit_period=off  period=1  block_type=tdd
      settings: infoedit=Samples presented at the input are selected and down-sampled according to the frame sampling pattern specified. The sampled input is presented either as a single or multiple channel at the output.  xl_area=[24 48 0 0 0 0 0]  block_version=9.1.01
  YA : Outport
  YB : Outport  Port=2
  wires:
  TDD/2 -> YB/1
  TDD/1 -> YA/1
  Adders/1(Out1) -> TDD/1
  Sample RAMs/8(Out8) -> Mults & ROMs/8(In8)
  Sample RAMs/7(Out7) -> Mults & ROMs/7(In7)
  Sample RAMs/6(Out6) -> Mults & ROMs/6(In6)
  Sample RAMs/5(Out5) -> Mults & ROMs/5(In5)
  Sample RAMs/4(Out4) -> Mults & ROMs/4(In4)
  Sample RAMs/3(Out3) -> Mults & ROMs/3(In3)
  Sample RAMs/2(Out2) -> Mults & ROMs/2(In2)
  Sample RAMs/1(Out1) -> Mults & ROMs/1(In1)
  XB/1 -> Sample RAMs/2(B)
  XA/1 -> Sample RAMs/1(A)
  Mults & ROMs/1(Out1) -> Adders/1(In1)
  Mults & ROMs/2(Out2) -> Adders/2(In2)
  Mults & ROMs/3(Out3) -> Adders/3(In3)
  Mults & ROMs/4(Out4) -> Adders/4(In4)
  Mults & ROMs/5(Out5) -> Adders/5(In5)
  Mults & ROMs/6(Out6) -> Adders/6(In6)
  Mults & ROMs/7(Out7) -> Adders/7(In7)
  Mults & ROMs/8(Out8) -> Adders/8(In8)

== system rate_change_filters_txrx_2ch/Tx Path/Chirp ==
  Chirp Signal : simulink/Sources/Chirp Signal  f1=0  T=512  f2=0.5
  Gain : Gain  Gain=0.95
  Out1 : Outport
  wires:
  Chirp Signal/1 -> Gain/1
  Gain/1 -> Out1/1

== system rate_change_filters_txrx_2ch/Tx Path/Chirp1 ==
  Chirp Signal : simulink/Sources/Chirp Signal  f1=0  T=512  f2=0.5
  Gain : Gain  Gain=-0.95
  Out1 : Outport
  wires:
  Gain/1 -> Out1/1
  Chirp Signal/1 -> Gain/1

== system rate_change_filters_txrx_2ch/Rx Path/2-Ch Decimation A/Adders ==
  In1 : Inport
  In2 : Inport  Port=2
  In3 : Inport  Port=3
  In4 : Inport  Port=4
  In5 : Inport  Port=5
  In6 : Inport  Port=6
  In7 : Inport  Port=7
  In8 : Inport  Port=8
  In9 : Inport  Port=9
  In10 : Inport  Port=10
  In11 : Inport  Port=11
  In12 : Inport  Port=12
  In13 : Inport  Port=13
  In14 : Inport  Port=14
  In15 : Inport  Port=15
  In16 : Inport  Port=16
  AddSub6 : xbsIndex_r4/AddSub  mode=Addition  use_carryin=off  use_carryout=off  en=off  latency=0  precision=Full  arith_type="Signed  (2's comp)"  n_bits=1  bin_pt=0  quantization=Truncate  overflow=Flag as error  dbl_ovrd=off  use_behavioral_HDL=on  hw_selection=Fabric  pipelined=off  use_rpm=on  block_type=addsub
      settings: xl_area=[15 0 0 28 0 0 0]  block_version=9.1.01
  Adder Tree : Subsystem
  Adder Tree1 : Subsystem
  Out1 : Outport
  wires:
  Adder Tree/1(Out1) -> AddSub6/2
  Adder Tree1/1(Out1) -> AddSub6/1
  In1/1 -> Adder Tree1/1(In1)
  In2/1 -> Adder Tree1/2(In2)
  In3/1 -> Adder Tree1/3(In3)
  In4/1 -> Adder Tree1/4(In4)
  In5/1 -> Adder Tree1/5(In5)
  In6/1 -> Adder Tree1/6(In6)
  In7/1 -> Adder Tree1/7(In7)
  In8/1 -> Adder Tree1/8(In8)
  In9/1 -> Adder Tree/1(In1)
  In10/1 -> Adder Tree/2(In2)
  In11/1 -> Adder Tree/3(In3)
  In12/1 -> Adder Tree/4(In4)
  AddSub6/1 -> Out1/1
  In13/1 -> Adder Tree/5(In5)
  In14/1 -> Adder Tree/6(In6)
  In15/1 -> Adder Tree/7(In7)
  In16/1 -> Adder Tree/8(In8)

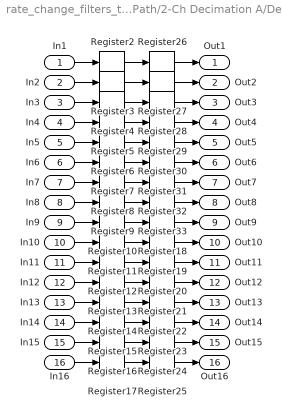
== system rate_change_filters_txrx_2ch/Rx Path/2-Ch Decimation A/Delays ==
  In1 : Inport
  In2 : Inport  Port=2
  In3 : Inport  Port=3
  In4 : Inport  Port=4
  In5 : Inport  Port=5
  In6 : Inport  Port=6
  In7 : Inport  Port=7
  In8 : Inport  Port=8
  In9 : Inport  Port=9
  In10 : Inport  Port=10
  In11 : Inport  Port=11
  In12 : Inport  Port=12
  In13 : Inport  Port=13
  In14 : Inport  Port=14
  In15 : Inport  Port=15
  In16 : Inport  Port=16
  Register{2..33} (32 alike) : xbsIndex_r4/Register  init=0  rst=off  en=off  dbl_ovrd=off  block_type=register
      settings: xl_area=[7 14 0 0 0 0 0]
  Out1 : Outport
  Out2 : Outport  Port=2
  Out3 : Outport  Port=3
  Out4 : Outport  Port=4
  Out5 : Outport  Port=5
  Out6 : Outport  Port=6
  Out7 : Outport  Port=7
  Out8 : Outport  Port=8
  Out9 : Outport  Port=9
  Out10 : Outport  Port=10
  Out11 : Outport  Port=11
  Out12 : Outport  Port=12
  Out13 : Outport  Port=13
  Out14 : Outport  Port=14
  Out15 : Outport  Port=15
  Out16 : Outport  Port=16
  wires:
  Register2/1 -> Register26/1
  Register3/1 -> Register27/1
  Register4/1 -> Register28/1
  Register5/1 -> Register29/1
  Register6/1 -> Register30/1
  Register7/1 -> Register31/1
  Register8/1 -> Register32/1
  Register9/1 -> Register33/1
  Register10/1 -> Register18/1
  Register11/1 -> Register19/1
  Register12/1 -> Register20/1
  Register13/1 -> Register21/1
  Register14/1 -> Register22/1
  Register15/1 -> Register23/1
  Register16/1 -> Register24/1
  Register17/1 -> Register25/1
  In1/1 -> Register2/1
  Register26/1 -> Out1/1
  Register27/1 -> Out2/1
  In2/1 -> Register3/1
  Register28/1 -> Out3/1
  In3/1 -> Register4/1
  Register29/1 -> Out4/1
  In4/1 -> Register5/1
  Register30/1 -> Out5/1
  In5/1 -> Register6/1
  Register31/1 -> Out6/1
  In6/1 -> Register7/1
  Register32/1 -> Out7/1
  In7/1 -> Register8/1
  Register33/1 -> Out8/1
  In8/1 -> Register9/1
  In9/1 -> Register10/1
  Register18/1 -> Out9/1
  In10/1 -> Register11/1
  Register19/1 -> Out10/1
  In11/1 -> Register12/1
  Register20/1 -> Out11/1
  In12/1 -> Register13/1
  Register21/1 -> Out12/1
  In13/1 -> Register14/1
  Register22/1 -> Out13/1
  In14/1 -> Register15/1
  Register23/1 -> Out14/1
  In15/1 -> Register16/1
  Register24/1 -> Out15/1
  In16/1 -> Register17/1
  Register25/1 -> Out16/1

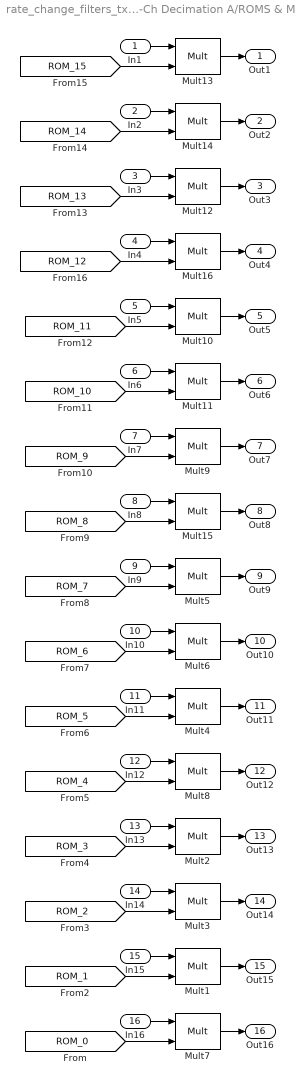
== system rate_change_filters_txrx_2ch/Rx Path/2-Ch Decimation A/ROMS & Mults ==
  In1 : Inport
  In2 : Inport  Port=2
  In3 : Inport  Port=3
  In4 : Inport  Port=4
  In5 : Inport  Port=5
  In6 : Inport  Port=6
  In7 : Inport  Port=7
  In8 : Inport  Port=8
  In9 : Inport  Port=9
  In10 : Inport  Port=10
  In11 : Inport  Port=11
  In12 : Inport  Port=12
  In13 : Inport  Port=13
  In14 : Inport  Port=14
  In15 : Inport  Port=15
  In16 : Inport  Port=16
  Mult{1..16} (16 alike) : xbsIndex_r4/Mult  precision=User Defined  arith_type="Signed  (2's comp)"  n_bits=24  bin_pt=22  quantization=Truncate  overflow=Flag as error  en=off  latency=1  dbl_ovrd=off  use_behavioral_HDL=off  opt=Speed  use_embedded=on  optimum_pipeline=off  pipeline=off  use_rpm=on  placement_style=Rectangular shape  block_type=mult
      settings: infoedit=Hardware notes: To use the internal pipeline stage of the dedicated multiplier you must select 'Pipeline for maximum performance'.  xl_area=[16 32 0 32 0 1 0]  block_version=9.1.01
  Out1 : Outport
  Out2 : Outport  Port=2
  Out3 : Outport  Port=3
  Out4 : Outport  Port=4
  Out5 : Outport  Port=5
  Out6 : Outport  Port=6
  Out7 : Outport  Port=7
  Out8 : Outport  Port=8
  Out9 : Outport  Port=9
  Out10 : Outport  Port=10
  Out11 : Outport  Port=11
  Out12 : Outport  Port=12
  Out13 : Outport  Port=13
  Out14 : Outport  Port=14
  Out15 : Outport  Port=15
  Out16 : Outport  Port=16
  wires:
  [ROM_15] -> Mult13/2
  [ROM_14] -> Mult14/2
  [ROM_13] -> Mult12/2
  [ROM_12] -> Mult16/2
  [ROM_11] -> Mult10/2
  [ROM_10] -> Mult11/2
  [ROM_9] -> Mult9/2
  [ROM_8] -> Mult15/2
  [ROM_7] -> Mult5/2
  [ROM_6] -> Mult6/2
  [ROM_5] -> Mult4/2
  [ROM_4] -> Mult8/2
  [ROM_3] -> Mult2/2
  [ROM_2] -> Mult3/2
  [ROM_1] -> Mult1/2
  [ROM_0] -> Mult7/2
  In1/1 -> Mult13/1
  Mult13/1 -> Out1/1
  In2/1 -> Mult14/1
  Mult14/1 -> Out2/1
  In3/1 -> Mult12/1
  Mult12/1 -> Out3/1
  In4/1 -> Mult16/1
  Mult16/1 -> Out4/1
  In5/1 -> Mult10/1
  Mult10/1 -> Out5/1
  In6/1 -> Mult11/1
  Mult11/1 -> Out6/1
  In7/1 -> Mult9/1
  Mult9/1 -> Out7/1
  In8/1 -> Mult15/1
  Mult15/1 -> Out8/1
  In9/1 -> Mult5/1
  Mult5/1 -> Out9/1
  In10/1 -> Mult6/1
  Mult6/1 -> Out10/1
  In11/1 -> Mult4/1
  Mult4/1 -> Out11/1
  In12/1 -> Mult8/1
  Mult8/1 -> Out12/1
  In13/1 -> Mult2/1
  Mult2/1 -> Out13/1
  In14/1 -> Mult3/1
  Mult3/1 -> Out14/1
  In15/1 -> Mult1/1
  Mult1/1 -> Out15/1
  In16/1 -> Mult7/1
  Mult7/1 -> Out16/1

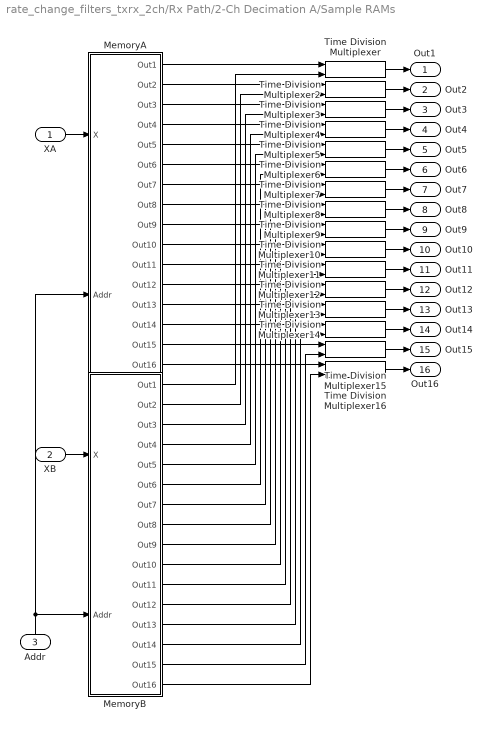
== system rate_change_filters_txrx_2ch/Rx Path/2-Ch Decimation A/Sample RAMs ==
  XA : Inport
  XB : Inport  Port=2
  Addr : Inport  Port=3
  MemoryA : Subsystem
  MemoryB : Subsystem
  Time Division Multiplexer{,2..16} (16 alike) : xbsIndex_r4/Time Division Multiplexer  inputs=2  vin=off  dbl_ovrd=off  explicit_period=off  period=1  block_type=tdm
      settings: infoedit="Multiple inputs are sampled and  presented serially at the output."  xl_area=[3 2 0 31 0 0 0]  block_version=10.1.3
  Out1 : Outport
  Out2 : Outport  Port=2
  Out3 : Outport  Port=3
  Out4 : Outport  Port=4
  Out5 : Outport  Port=5
  Out6 : Outport  Port=6
  Out7 : Outport  Port=7
  Out8 : Outport  Port=8
  Out9 : Outport  Port=9
  Out10 : Outport  Port=10
  Out11 : Outport  Port=11
  Out12 : Outport  Port=12
  Out13 : Outport  Port=13
  Out14 : Outport  Port=14
  Out15 : Outport  Port=15
  Out16 : Outport  Port=16
  wires:
  Addr/1 -> MemoryA/2(Addr), MemoryB/2(Addr)
  MemoryA/1(Out1) -> Time Division Multiplexer/1
  MemoryA/2(Out2) -> Time Division Multiplexer2/1
  MemoryA/3(Out3) -> Time Division Multiplexer3/1
  MemoryA/4(Out4) -> Time Division Multiplexer4/1
  MemoryA/5(Out5) -> Time Division Multiplexer5/1
  MemoryA/6(Out6) -> Time Division Multiplexer6/1
  MemoryA/7(Out7) -> Time Division Multiplexer7/1
  MemoryA/8(Out8) -> Time Division Multiplexer8/1
  MemoryA/9(Out9) -> Time Division Multiplexer9/1
  MemoryA/10(Out10) -> Time Division Multiplexer10/1
  MemoryA/11(Out11) -> Time Division Multiplexer11/1
  MemoryA/12(Out12) -> Time Division Multiplexer12/1
  MemoryA/13(Out13) -> Time Division Multiplexer13/1
  MemoryA/14(Out14) -> Time Division Multiplexer14/1
  MemoryA/15(Out15) -> Time Division Multiplexer15/1
  MemoryA/16(Out16) -> Time Division Multiplexer16/1
  MemoryB/1(Out1) -> Time Division Multiplexer/2
  MemoryB/2(Out2) -> Time Division Multiplexer2/2
  MemoryB/3(Out3) -> Time Division Multiplexer3/2
  MemoryB/4(Out4) -> Time Division Multiplexer4/2
  MemoryB/5(Out5) -> Time Division Multiplexer5/2
  MemoryB/6(Out6) -> Time Division Multiplexer6/2
  MemoryB/7(Out7) -> Time Division Multiplexer7/2
  MemoryB/8(Out8) -> Time Division Multiplexer8/2
  MemoryB/9(Out9) -> Time Division Multiplexer9/2
  MemoryB/10(Out10) -> Time Division Multiplexer10/2
  MemoryB/11(Out11) -> Time Division Multiplexer11/2
  MemoryB/12(Out12) -> Time Division Multiplexer12/2
  MemoryB/13(Out13) -> Time Division Multiplexer13/2
  MemoryB/14(Out14) -> Time Division Multiplexer14/2
  MemoryB/15(Out15) -> Time Division Multiplexer15/2
  MemoryB/16(Out16) -> Time Division Multiplexer16/2
  Time Division Multiplexer/1 -> Out1/1
  Time Division Multiplexer2/1 -> Out2/1
  Time Division Multiplexer3/1 -> Out3/1
  Time Division Multiplexer4/1 -> Out4/1
  XA/1 -> MemoryA/1(X)
  Time Division Multiplexer5/1 -> Out5/1
  Time Division Multiplexer6/1 -> Out6/1
  Time Division Multiplexer7/1 -> Out7/1
  Time Division Multiplexer8/1 -> Out8/1
  Time Division Multiplexer9/1 -> Out9/1
  Time Division Multiplexer10/1 -> Out10/1
  Time Division Multiplexer11/1 -> Out11/1
  Time Division Multiplexer12/1 -> Out12/1
  Time Division Multiplexer13/1 -> Out13/1
  Time Division Multiplexer14/1 -> Out14/1
  Time Division Multiplexer15/1 -> Out15/1
  Time Division Multiplexer16/1 -> Out16/1
  XB/1 -> MemoryB/1(X)

== system rate_change_filters_txrx_2ch/Rx Path/2-Ch Decimation B/Adders ==
  In1 : Inport
  In2 : Inport  Port=2
  In3 : Inport  Port=3
  In4 : Inport  Port=4
  In5 : Inport  Port=5
  In6 : Inport  Port=6
  In7 : Inport  Port=7
  In8 : Inport  Port=8
  In9 : Inport  Port=9
  In10 : Inport  Port=10
  In11 : Inport  Port=11
  In12 : Inport  Port=12
  In13 : Inport  Port=13
  In14 : Inport  Port=14
  In15 : Inport  Port=15
  In16 : Inport  Port=16
  AddSub6 : xbsIndex_r4/AddSub  mode=Addition  use_carryin=off  use_carryout=off  en=off  latency=0  precision=Full  arith_type="Signed  (2's comp)"  n_bits=1  bin_pt=0  quantization=Truncate  overflow=Flag as error  dbl_ovrd=off  use_behavioral_HDL=on  hw_selection=Fabric  pipelined=off  use_rpm=on  block_type=addsub
      settings: xl_area=[15 0 0 28 0 0 0]  block_version=9.1.01
  Adder Tree : Subsystem
  Adder Tree1 : Subsystem
  Out1 : Outport
  wires:
  In16/1 -> Adder Tree/8(In8)
  In15/1 -> Adder Tree/7(In7)
  In14/1 -> Adder Tree/6(In6)
  In13/1 -> Adder Tree/5(In5)
  AddSub6/1 -> Out1/1
  In12/1 -> Adder Tree/4(In4)
  In11/1 -> Adder Tree/3(In3)
  In10/1 -> Adder Tree/2(In2)
  In9/1 -> Adder Tree/1(In1)
  In8/1 -> Adder Tree1/8(In8)
  In7/1 -> Adder Tree1/7(In7)
  In6/1 -> Adder Tree1/6(In6)
  In5/1 -> Adder Tree1/5(In5)
  In4/1 -> Adder Tree1/4(In4)
  In3/1 -> Adder Tree1/3(In3)
  In2/1 -> Adder Tree1/2(In2)
  In1/1 -> Adder Tree1/1(In1)
  Adder Tree1/1(Out1) -> AddSub6/1
  Adder Tree/1(Out1) -> AddSub6/2
